simulink model "plantaCPC"  (R2026a)
settings: Solver=ode4  StopTime=inf  EnableMultiTasking=on
values from neighbouring files (symbols this model uses):
  A = 0.159    [parametros.m]    (also in prbs_calc_L3.m; ti_calc.m)
  a1 = (a11 + a12)/2    [areas.m]    (also in parametros.m = 0.0006136)
  a2 = mean([a21 a22],2)    [areas.m]    (also in parametros.m = 0.00054678)
  a3 = mean([a31 a32],2)    [areas.m]    (also in parametros.m = 0.00035752; prbs_calc_L3.m = 0.00035752; ti_calc.m = 0.00035752)
  a4 = mean([a41 a42],2)    [areas.m]    (also in parametros.m = 0.0004182; ti_calc.m = 0.0004182)
  gamma1 = 0.455    [areas.m]    (also in parametros.m)
  gamma2 = 0.4195    [areas.m]    (also in parametros.m)
  k1 = q_max    (= 0.0017)    [areas.m]    (also in parametros.m)
  k2 = q_max    (= 0.0017)    [areas.m]    (also in parametros.m)
libraries: simulink x16, opcualib x2
settings Model: Creator=Administrator  LastModifiedBy=agusc
settings DebuggingCC: UnderspecifiedInitializationDetection=Classic
settings HardwareCC: ProdHWDeviceType=32-bit Generic

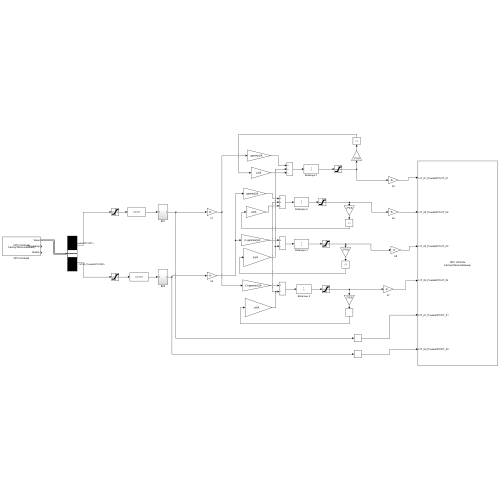
[thumbnail: Simulink's stored preview of the top-level diagram]
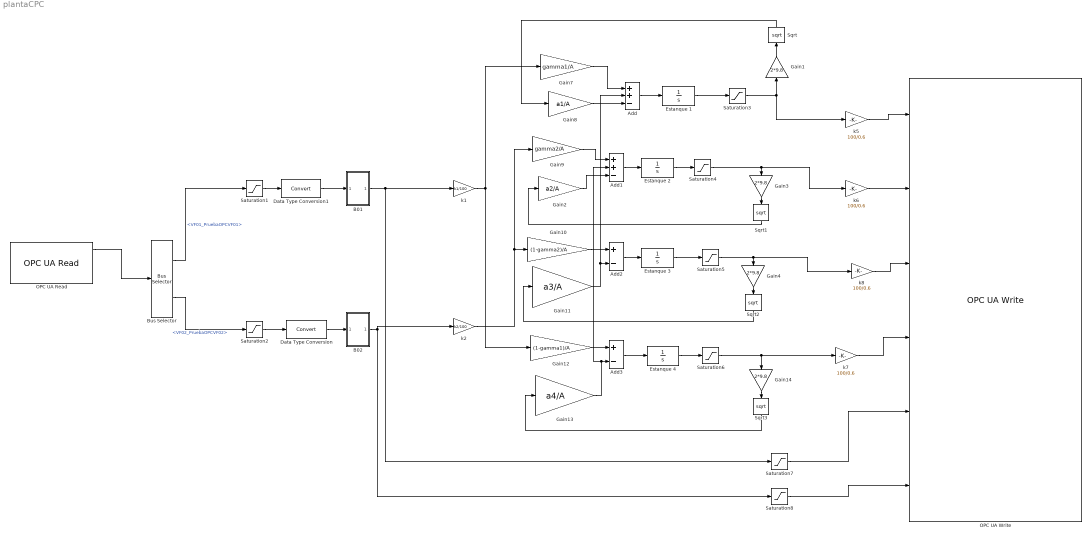
== system plantaCPC ==
  Add : Sum  Inputs=++-
  Add1 : Sum  Inputs=++-
  Add2 : Sum  Inputs=+-
  Add3 : Sum  Inputs=+-
  B01 : Subsystem
  B02 : Subsystem
  Bus Selector : BusSelector  OutputSignals=VF01_PruebaOPCVF01,VF02_PruebaOPCVF02
  Data Type Conversion : DataTypeConversion  SaturateOnIntegerOverflow=off  RndMeth=Floor
  Data Type Conversion1 : DataTypeConversion  SaturateOnIntegerOverflow=off  RndMeth=Floor
  Estanque 1 : TransferFcn  Denominator=[1 0]
  "Estanque 2 " : TransferFcn  Denominator=[1 0]
  Estanque 3 : TransferFcn  Denominator=[1 0]
  Estanque 4 : TransferFcn  Denominator=[1 0]
  Gain{1,3..4,14} (4 alike) : Gain  Gain=2*9.8
  Gain10 : Gain  Gain=(1-gamma2)/A
  Gain11 : Gain  Gain=a3/A
  Gain12 : Gain  Gain=(1-gamma1)/A
  Gain13 : Gain  Gain=a4/A
  Gain2 : Gain  Gain=a2/A
  Gain7 : Gain  Gain=gamma1/A
  Gain8 : Gain  Gain=a1/A
  Gain9 : Gain  Gain=gamma2/A
  OPC UA Read : opcualib/OPC UA Read  SelectedServer=FactoryTalkLinxGateway  ServerList=FactoryTalkLinxGateway  NodeList={ '1', 'VF01', '2', '[Prueba OPC]VF01', 'off'; '2', 'VF02', '2', '[Prueba OPC]VF02', 'off' }  ShowQualityPort=on  ShowTimestampPort=on  ShowTimestampPortAs=Seconds since start  SampleTime=-1
  OPC UA Write : opcualib/OPC UA Write  SelectedServer=FactoryTalkLinxGateway  ServerList=FactoryTalkLinxGateway  SampleTime=-1  NodeList={ '1', 'LIT_01', '2', '[Prueba OPC]LIT_01', 'off'; '2', 'LIT_02', '2', '[Prueba OPC]LIT_02', 'off'; '3', 'LIT_03', '2', '[Prueba OPC]LIT_03', 'off'; '4', 'LIT_04', '2', '[Prueba OPC]LIT_04', 'off'; '5', 'FIT_01', '2', '[Prueba OPC]FIT_01', 'off'; '6', 'FIT_02', '2', '[Prueba OPC]FIT_02', 'off' }
  Saturation{1..2,7..8} (4 alike) : Saturate  UpperLimit=100  LowerLimit=0
  Saturation{3..6} (4 alike) : Saturate  UpperLimit=0.8  LowerLimit=0
  Sqrt{,1..3} (4 alike) : Sqrt
  k1 : Gain  Gain=k1/100
  k2 : Gain  Gain=k2/100
  k{5..8} (4 alike) : Gain  Gain=100/0.6
  wires:
  Saturation3/1 -> k5/1, Gain1/1
  Saturation4/1 -> k6/1, Gain3/1
  Saturation5/1 -> k8/1, Gain4/1
  Estanque 1/1 -> Saturation3/1
  "Estanque 2 "/1 -> Saturation4/1
  Estanque 4/1 -> Saturation6/1
  Saturation2/1 -> Data Type Conversion/1
  Saturation1/1 -> Data Type Conversion1/1
  B01/1(Out1) -> Saturation7/1, k1/1
  B02/1(Out1) -> k2/1, Saturation8/1
  Gain7/1 -> Add/1
  k1/1 -> Gain7/1, Gain12/1
  Gain8/1 -> Add/3
  Add/1 -> Estanque 1/1
  Add1/1 -> "Estanque 2 "/1
  Add2/1 -> Estanque 3/1
  Add3/1 -> Estanque 4/1
  Gain9/1 -> Add1/1
  k2/1 -> Gain9/1, Gain10/1
  Gain2/1 -> Add1/3
  Gain10/1 -> Add2/1
  Gain11/1 -> Add/2, Add2/2
  Gain12/1 -> Add3/1
  Gain13/1 -> Add1/2, Add3/2
  Estanque 3/1 -> Saturation5/1
  Gain1/1 -> Sqrt/1
  Sqrt/1 -> Gain8/1
  Gain3/1 -> Sqrt1/1
  Sqrt1/1 -> Gain2/1
  Gain4/1 -> Sqrt2/1
  Gain14/1 -> Sqrt3/1
  Saturation6/1 -> Gain14/1, k7/1
  Sqrt3/1 -> Gain13/1
  Sqrt2/1 -> Gain11/1
  OPC UA Read/1 -> Bus Selector/1
  Data Type Conversion/1 -> B02/1(In1)
  Data Type Conversion1/1 -> B01/1(In1)
  Bus Selector/1 -> Saturation1/1  "<VF01_PruebaOPCVF01>"
  Bus Selector/2 -> Saturation2/1  "<VF02_PruebaOPCVF02>"
  Saturation7/1 -> OPC UA Write/5
  Saturation8/1 -> OPC UA Write/6
  k8/1 -> OPC UA Write/3
  k6/1 -> OPC UA Write/2
  k5/1 -> OPC UA Write/1
  k7/1 -> OPC UA Write/4

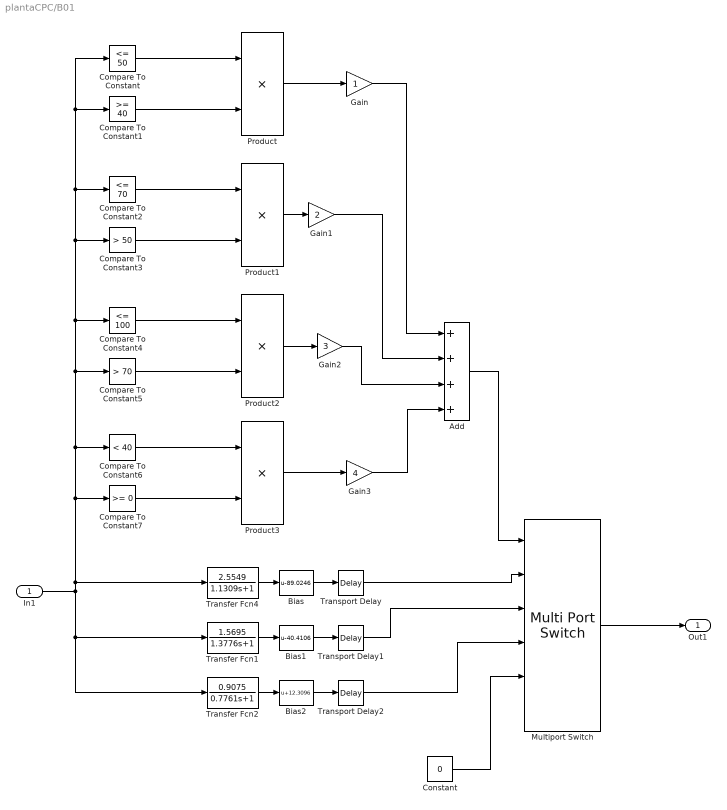
== system plantaCPC/B01 ==
  In1 : Inport
  Add : Sum  Inputs=++++
  Bias : Bias  Bias=-89.0246  SaturateOnIntegerOverflow=off
  Bias1 : Bias  Bias=-40.4106  SaturateOnIntegerOverflow=off
  Bias2 : Bias  Bias=12.3096  SaturateOnIntegerOverflow=off
  Compare To Constant : simulink/Logic and Bit Operations/Compare To Constant  relop=<=  const=50  OutDataTypeStr=boolean
  Compare To Constant1 : simulink/Logic and Bit Operations/Compare To Constant  relop=>=  const=40  OutDataTypeStr=boolean
  Compare To Constant2 : simulink/Logic and Bit Operations/Compare To Constant  relop=<=  const=70  OutDataTypeStr=boolean
  Compare To Constant3 : simulink/Logic and Bit Operations/Compare To Constant  relop=>  const=50  OutDataTypeStr=boolean
  Compare To Constant4 : simulink/Logic and Bit Operations/Compare To Constant  relop=<=  const=100  OutDataTypeStr=boolean
  Compare To Constant5 : simulink/Logic and Bit Operations/Compare To Constant  relop=>  const=70  OutDataTypeStr=boolean
  Compare To Constant6 : simulink/Logic and Bit Operations/Compare To Constant  relop=<  const=40  OutDataTypeStr=boolean
  Compare To Constant7 : simulink/Logic and Bit Operations/Compare To Constant  relop=>=  const=0  OutDataTypeStr=boolean
  Constant : Constant  Value=0
  Gain : Gain
  Gain1 : Gain  Gain=2
  Gain2 : Gain  Gain=3
  Gain3 : Gain  Gain=4
  Multiport Switch : MultiPortSwitch  Inputs=5  SaturateOnIntegerOverflow=off  InputSameDT=off
  Product{,1..3} (4 alike) : Product
  Transfer Fcn1 : TransferFcn  Numerator=[1.5695]  Denominator=[1.3776 1]
  Transfer Fcn2 : TransferFcn  Numerator=[0.9075]  Denominator=[0.7761 1]
  Transfer Fcn4 : TransferFcn  Numerator=[2.5549]  Denominator=[1.1309 1]
  Transport Delay : TransportDelay  DelayTime=0.6
  Transport Delay1 : TransportDelay  DelayTime=0.5
  Transport Delay2 : TransportDelay  DelayTime=0.5
  Out1 : Outport
  wires:
  Multiport Switch/1 -> Out1/1
  Product/1 -> Gain/1
  Gain/1 -> Add/1
  Product1/1 -> Gain1/1
  Gain1/1 -> Add/2
  Gain2/1 -> Add/3
  Product2/1 -> Gain2/1
  Add/1 -> Multiport Switch/1
  Compare To Constant/1 -> Product/1
  Transfer Fcn4/1 -> Bias/1
  Transfer Fcn1/1 -> Bias1/1
  Transfer Fcn2/1 -> Bias2/1
  Compare To Constant1/1 -> Product/2
  Compare To Constant2/1 -> Product1/1
  Compare To Constant3/1 -> Product1/2
  Compare To Constant4/1 -> Product2/1
  Compare To Constant5/1 -> Product2/2
  Transport Delay/1 -> Multiport Switch/2
  Transport Delay1/1 -> Multiport Switch/3
  Transport Delay2/1 -> Multiport Switch/4
  Bias/1 -> Transport Delay/1
  Bias1/1 -> Transport Delay1/1
  Bias2/1 -> Transport Delay2/1
  Product3/1 -> Gain3/1
  Compare To Constant6/1 -> Product3/1
  Compare To Constant7/1 -> Product3/2
  In1/1 -> Compare To Constant7/1, Compare To Constant6/1, Compare To Constant4/1, Compare To Constant2/1, Compare To Constant1/1, Compare To Constant/1, Compare To Constant3/1, Compare To Constant5/1, Transfer Fcn4/1, Transfer Fcn2/1, Transfer Fcn1/1
  Gain3/1 -> Add/4
  Constant/1 -> Multiport Switch/5

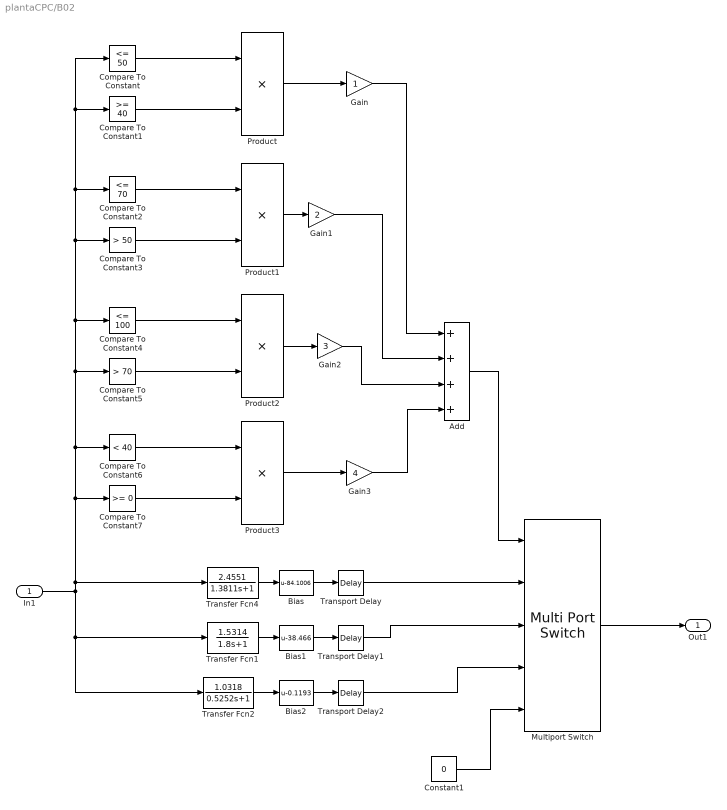
== system plantaCPC/B02 ==
  In1 : Inport
  Add : Sum  Inputs=++++
  Bias : Bias  Bias=-84.1006  SaturateOnIntegerOverflow=off
  Bias1 : Bias  Bias=-38.466  SaturateOnIntegerOverflow=off
  Bias2 : Bias  Bias=-0.1193  SaturateOnIntegerOverflow=off
  Compare To Constant : simulink/Logic and Bit Operations/Compare To Constant  relop=<=  const=50  OutDataTypeStr=boolean
  Compare To Constant1 : simulink/Logic and Bit Operations/Compare To Constant  relop=>=  const=40  OutDataTypeStr=boolean
  Compare To Constant2 : simulink/Logic and Bit Operations/Compare To Constant  relop=<=  const=70  OutDataTypeStr=boolean
  Compare To Constant3 : simulink/Logic and Bit Operations/Compare To Constant  relop=>  const=50  OutDataTypeStr=boolean
  Compare To Constant4 : simulink/Logic and Bit Operations/Compare To Constant  relop=<=  const=100  OutDataTypeStr=boolean
  Compare To Constant5 : simulink/Logic and Bit Operations/Compare To Constant  relop=>  const=70  OutDataTypeStr=boolean
  Compare To Constant6 : simulink/Logic and Bit Operations/Compare To Constant  relop=<  const=40  OutDataTypeStr=boolean
  Compare To Constant7 : simulink/Logic and Bit Operations/Compare To Constant  relop=>=  const=0  OutDataTypeStr=boolean
  Constant1 : Constant  Value=0
  Gain : Gain
  Gain1 : Gain  Gain=2
  Gain2 : Gain  Gain=3
  Gain3 : Gain  Gain=4
  Multiport Switch : MultiPortSwitch  Inputs=4  SaturateOnIntegerOverflow=off  InputSameDT=off
  Product{,1..3} (4 alike) : Product
  Transfer Fcn1 : TransferFcn  Numerator=[1.5314]  Denominator=[1.8 1]
  Transfer Fcn2 : TransferFcn  Numerator=[1.0318]  Denominator=[0.5252 1]
  Transfer Fcn4 : TransferFcn  Numerator=[2.4551]  Denominator=[1.3811 1]
  Transport Delay : TransportDelay  DelayTime=0.5
  Transport Delay1 : TransportDelay  DelayTime=0.5
  Transport Delay2 : TransportDelay  DelayTime=0.8
  Out1 : Outport
  wires:
  Multiport Switch/1 -> Out1/1
  Product/1 -> Gain/1
  Gain/1 -> Add/1
  Product1/1 -> Gain1/1
  Gain1/1 -> Add/2
  Gain2/1 -> Add/3
  Product2/1 -> Gain2/1
  Add/1 -> Multiport Switch/1
  Compare To Constant/1 -> Product/1
  Transfer Fcn4/1 -> Bias/1
  Transfer Fcn1/1 -> Bias1/1
  Transfer Fcn2/1 -> Bias2/1
  Compare To Constant1/1 -> Product/2
  Compare To Constant2/1 -> Product1/1
  Compare To Constant3/1 -> Product1/2
  Compare To Constant4/1 -> Product2/1
  Compare To Constant5/1 -> Product2/2
  Transport Delay/1 -> Multiport Switch/2
  Transport Delay1/1 -> Multiport Switch/3
  Transport Delay2/1 -> Multiport Switch/4
  Bias/1 -> Transport Delay/1
  Bias1/1 -> Transport Delay1/1
  Bias2/1 -> Transport Delay2/1
  Product3/1 -> Gain3/1
  Compare To Constant6/1 -> Product3/1
  Compare To Constant7/1 -> Product3/2
  In1/1 -> Compare To Constant7/1, Compare To Constant6/1, Compare To Constant4/1, Compare To Constant2/1, Compare To Constant1/1, Compare To Constant/1, Compare To Constant3/1, Compare To Constant5/1, Transfer Fcn4/1, Transfer Fcn2/1, Transfer Fcn1/1
  Gain3/1 -> Add/4
  Constant1/1 -> Multiport Switch/5
